simulink model "original"  (R2018a)
settings: Solver=VariableStepAuto  StartTime=0.0  StopTime=10.0  RelTol=1e-3
undefined symbols (not defined in the file): DiscIntNeverNeededParam, sigbuilder_block
libraries: simulink x479
(part 1 of 9)
settings Model: Creator=cyfuzz  LastModifiedBy=ishaf
settings CodeAppCC: StateflowObjectComments=on

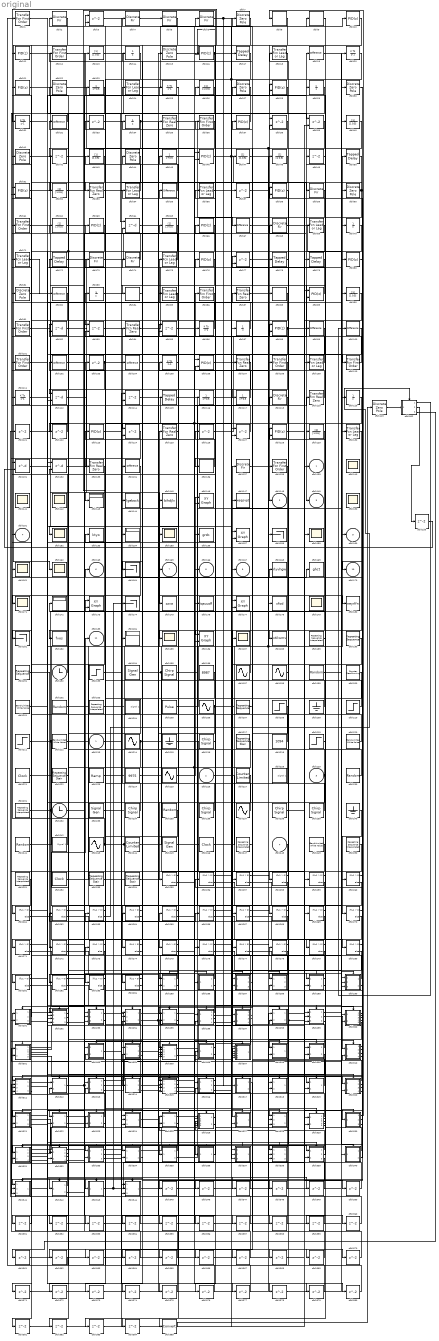
== system original ==
  cfblk213 : Inport
  cfblk226 : Inport  Port=2
  cfblk229 : Inport  Port=3
  cfblk248 : Inport  Port=4
  cfblk{1,12,36,61,86,91,101,108,110,138} (10 alike) : simulink/Discrete/Transfer Fcn First Order  PoleZ=0.95  ICPrevOutput=0.0  DoSatur=off
      settings: SourceProductName=Simulink
  cfblk{10..11,16,21,37,63,66,76,80,123} (10 alike) : simulink/Continuous/PID Controller  Controller=PID  TimeDomain=Discrete-time  SampleTime=1  IntegratorMethod=Forward Euler  FilterMethod=Forward Euler  Form=Parallel  UseFilter=on  ControllerParametersSource=internal  P=1  I=1  D=0  N=100  InitialConditionSource=internal  InitialConditionForIntegrator=0  InitialConditionForFilter=0  ExternalReset=none  LimitOutput=off  UpperSaturationLimit=inf  LowerSaturationLimit=-inf  LinearizeAsGain=off  AntiWindupMode=none  Kb=1  TrackingMode=off  Kt=1  PParamMin=[]  PParamMax=[]  IParamMin=[]  IParamMax=[]  DParamMin=[]  DParamMax=[]  NParamMin=[]  NParamMax=[]  KbParamMin=[]  KbParamMax=[]  KtParamMin=[]  KtParamMax=[]  POutMin=[]  POutMax=[]  IOutMin=[]  IOutMax=[]  DOutMin=[]  DOutMax=[]  NOutMin=[]  NOutMax=[]  KbOutMin=[]  KbOutMax=[]  KtOutMin=[]  KtOutMax=[]  IntegratorOutMin=[]  IntegratorOutMax=[]  FilterOutMin=[]  FilterOutMax=[]  SumOutMin=[]  SumOutMax=[]  SumI1OutMin=[]  SumI1OutMax=[]  SumI2OutMin=[]  SumI2OutMax=[]  SumI3OutMin=[]  SumI3OutMax=[]  SumDOutMin=[]  SumDOutMax=[]  SaturationOutMin=[]  SaturationOutMax=[]  IntegratorContinuousStateAttributes=''  IntegratorStateMustResolveToSignalObject=off  IntegratorRTWStateStorageClass=Auto  FilterContinuousStateAttributes=''  FilterStateMustResolveToSignalObject=off  FilterRTWStateStorageClass=Auto  DifferentiatorICPrevScaledInput=0  DifferentiatorOutMin=[]  DifferentiatorOutMax=[]  FilterDiffOutCoefMin=[]  FilterDiffOutCoefMax=[]  SumDenOutMin=[]  SumDenOutMax=[]  SumNumOutMin=[]  SumNumOutMax=[]  ReciprocalOutMin=[]  ReciprocalOutMax=[]  DivideOutMin=[]  DivideOutMax=[]  TunerSelectOption=Transfer Function Based (PID Tuner App)
  cfblk{19,32,55,67,82,99..100,102,104,134} (10 alike) : simulink/Discrete/Difference  ICPrevInput=0.0  OutMin=[]  OutMax=[]  OutDataTypeStr=Inherit: Inherit via back propagation  OutDataType=fixdt(1, 16)  OutScaling=2^-10  DoSatur=off
  cfblk{33,42,49,57,103,121..122,126,135,345..384} (49 alike) : Delay  SampleTime=1
  cfblk{20,25,31,96,105,111} (6 alike) : DiscreteIntegrator  ICPrevOutput=DiscIntNeverNeededParam  ICPrevScaledInput=DiscIntNeverNeededParam
  cfblk{28,46,51,58,89,98,106,128} (8 alike) : simulink/Continuous/PID Controller (2DOF)  Controller=PID  TimeDomain=Discrete-time  SampleTime=1  IntegratorMethod=Forward Euler  FilterMethod=Forward Euler  Form=Parallel  UseFilter=on  ControllerParametersSource=internal  P=1  I=1  D=0  N=100  b=1  c=1  InitialConditionSource=internal  InitialConditionForIntegrator=0  InitialConditionForFilter=0  ExternalReset=none  LimitOutput=off  UpperSaturationLimit=inf  LowerSaturationLimit=-inf  LinearizeAsGain=off  AntiWindupMode=none  Kb=1  TrackingMode=off  Kt=1  PParamMin=[]  PParamMax=[]  IParamMin=[]  IParamMax=[]  DParamMin=[]  DParamMax=[]  NParamMin=[]  NParamMax=[]  bParamMin=[]  bParamMax=[]  cParamMin=[]  cParamMax=[]  KbParamMin=[]  KbParamMax=[]  KtParamMin=[]  KtParamMax=[]  POutMin=[]  POutMax=[]  IOutMin=[]  IOutMax=[]  DOutMin=[]  DOutMax=[]  NOutMin=[]  NOutMax=[]  bOutMin=[]  bOutMax=[]  cOutMin=[]  cOutMax=[]  KbOutMin=[]  KbOutMax=[]  KtOutMin=[]  KtOutMax=[]  IntegratorOutMin=[]  IntegratorOutMax=[]  FilterOutMin=[]  FilterOutMax=[]  SumOutMin=[]  SumOutMax=[]  Sum1OutMin=[]  Sum1OutMax=[]  Sum2OutMin=[]  Sum2OutMax=[]  Sum3OutMin=[]  Sum3OutMax=[]  SumI1OutMin=[]  SumI1OutMax=[]  SumI2OutMin=[]  SumI2OutMax=[]  SumI3OutMin=[]  SumI3OutMax=[]  SumDOutMin=[]  SumDOutMax=[]  SaturationOutMin=[]  SaturationOutMax=[]  IntegratorContinuousStateAttributes=''  IntegratorStateMustResolveToSignalObject=off  IntegratorRTWStateStorageClass=Auto  FilterContinuousStateAttributes=''  FilterStateMustResolveToSignalObject=off  FilterRTWStateStorageClass=Auto  DifferentiatorICPrevScaledInput=0  DifferentiatorOutMin=[]  DifferentiatorOutMax=[]  FilterDiffOutCoefMin=[]  FilterDiffOutCoefMax=[]  SumDenOutMin=[]  SumDenOutMax=[]  SumNumOutMin=[]  SumNumOutMax=[]  ReciprocalOutMin=[]  ReciprocalOutMax=[]  DivideOutMin=[]  DivideOutMax=[]  TunerSelectOption=Transfer Function Based (PID Tuner App)
  cfblk{35,53,87,94,107,119,125,133} (8 alike) : simulink/Discrete/Transfer Fcn Real Zero  ZeroZ=0.75  ICPrevInput=0.0  DoSatur=off
      settings: SourceProductName=Simulink  SourceProductBaseCode=SL
  cfblk{18,24,54,56,69,71,75,85,109,130} (10 alike) : simulink/Discrete/Transfer Fcn Lead or Lag  PoleZ=0.95  ZeroZ=0.75  ICPrevOutput=0.0  ICPrevInput=0.0  DoSatur=off
      settings: SourceProductName=Simulink  SourceProductBaseCode=SL
  cfblk{64,92,112,131..132} (5 alike) : Delay  DelayLengthSource=Input port  SampleTime=1
      settings: InputPortMap=u0,p1
  cfblk{7,15,22,27,30,41,44,60,81,113} (10 alike) : DiscreteZeroPole  Poles=[0 0.5]  Gain=1
  cfblk{3,38..39,77,93,95,114,124,127} (9 alike) : Delay  ShowEnablePort=on  SampleTime=1
      settings: InputPortMap=u0,e6
  cfblk{17,50,72,78..79,115} (6 alike) : simulink/Discrete/Tapped Delay  vinit=0.0  samptime=-1  NumDelays=1  DelayOrder=Oldest  includeCurrent=off
  cfblk{23,45,116..117} (4 alike) : DiscreteTransferFcn  SampleTime=1
  cfblk{2,4..6,59,68,73..74,118,137} (10 alike) : DiscreteFir  SampleTime=1
  cfblk{14,29,34,70,83,97,120} (7 alike) : UnitDelay
  cfblk{13,26,40,43,47..48,52,62,65,90,129} (11 alike) : DiscreteFilter  SampleTime=1
  cfblk{8..9,84,88,136} (5 alike) : DiscreteStateSpace
  cfblk{140..142,150,152,155,159,161..162,171,179,185,187} (13 alike) : Scope
      cfblk140 settings: Floating=on
      cfblk141 settings: Floating=on
      cfblk142 settings: Floating=on
      cfblk150 settings: Floating=on
      cfblk179 settings: Floating=on
  cfblk{143,154,172,184} (4 alike) : Display
  cfblk144 : ToWorkspace  VariableName=lgebsck  SaveFormat=Timeseries  SampleTime=-1
  cfblk145 : ToWorkspace  VariableName=bihdjlv  SaveFormat=Timeseries  SampleTime=-1
  cfblk{146,157,173,177,186} (5 alike) : simulink/Sinks/XY Graph  xmin=-1  xmax=1  ymin=-1  ymax=1  st=-1
  cfblk147 : ToWorkspace  VariableName=xeqpvpt  SaveFormat=Timeseries  SampleTime=-1
  cfblk153 : ToFile  Filename=ktyo  SaveFormat=Timeseries
  cfblk156 : ToFile  Filename=grzb  SaveFormat=Timeseries
  cfblk{158,164,174,181} (4 alike) : Terminator
  cfblk168 : ToWorkspace  VariableName=rlyvhgw  SaveFormat=Timeseries  SampleTime=-1
  cfblk169 : ToFile  Filename=ghct  SaveFormat=Timeseries
  cfblk175 : ToFile  Filename=zzva  SaveFormat=Timeseries
  cfblk176 : ToWorkspace  VariableName=iqauudf  SaveFormat=Timeseries  SampleTime=-1
  cfblk178 : ToFile  Filename=xfod  SaveFormat=Timeseries
  cfblk180 : ToWorkspace  VariableName=neyrlfn  SaveFormat=Timeseries  SampleTime=-1
  cfblk182 : ToFile  Filename=fvos  SaveFormat=Timeseries
  cfblk188 : ToWorkspace  VariableName=xtilwmv  SaveFormat=Timeseries  SampleTime=-1
  cfblk{189,203,231,247,250..251} (6 alike) : simulink/Sources/Repeating Sequence Interpolated  OutValues=[3 1 4 2 1].'  TimeValues=[0 0.1 0.5 0.6 1].'  LookUpMeth=Interpolation-Use End Values  tsamp=0.01  OutMin=[]  OutMax=[]  OutDataTypeStr=double  OutputDataTypeScalingMode=double  OutDataType=fixdt(0,8)  OutScaling=2^-10
  cfblk190 : simulink/Sources/Repeating Sequence  rep_seq_t=[0 2]  rep_seq_y=[0 2]
  cfblk191 : simulink/Sources/Repeating Sequence  rep_seq_t=[0 2]  rep_seq_y=[0 2]
  cfblk192 : Clock
  cfblk193 : Step  After=18  SampleTime=0
  cfblk194 : SignalGenerator  Units=rad/sec
  cfblk{195,216,234,236,238..239} (6 alike) : simulink/Sources/Chirp Signal  f1=0.1  T=100  f2=1
  cfblk196 : Constant  Value=8987
  cfblk{197..198,206,214,225,237,243} (7 alike) : Sin  SampleTime=0
  cfblk{199,230,235,241} (4 alike) : RandomNumber  SampleTime=0.1
  cfblk200 : simulink/Sources/Counter Free-Running  NumBits=16  tsamp=-1
  cfblk{201,212,220,249} (4 alike) : simulink/Sources/Band-Limited White Noise  Cov=[0.1]  Ts=0.1  seed=[23341]
  cfblk202 : UniformRandomNumber  SampleTime=0.1
  cfblk204 : Subsystem  Tag=STV Subsys  LoadFcn=sigbuilder_block('load');  StartFcn=sigbuilder_block('start');  StopFcn=sigbuilder_block('stop');  ClipboardFcn=sigbuilder_block('clipboard');  mask(Sigbuilder block){tuvar=[0:10]}
      mask help: Simulink:masks:SigbuilderBlock_MD
      mask init:
      | if ~strcmp(get_param(bdroot(gcbh),'SimulationStatus'),'stopped') tuvar = sigbuilder_block('maskInit'); end
      settings: CopyFcn=sigbuilder_block('copy');  DeleteFcn=sigbuilder_block('delete');  ModelCloseFcn=sigbuilder_block('modelClose');  PreSaveFcn=sigbuilder_block('preSave');  PauseFcn=sigbuilder_block('pause');  ContinueFcn=sigbuilder_block('continue');  NameChangeFcn=sigbuilder_block('namechange');  OpenFcn=sigbuilder_block('open',[437.6 199.2 550.4 400 ]);  CloseFcn=sigbuilder_block('close');
      mask Display: plot(0, 0, 100, 100,[2, 2, 32, 32, 2], [68, 8, 8, 68, 68],[32, 2], [38, 38], [32, 19, 2],[53, 60, 44], [32, 17, 17, 2],[16, 16, 31, 31]);txt = getActiveGroup(gcbh);text(2, 100, txt,'verticalAlignment', 'top');
  cfblk205 : DiscretePulseGenerator  PulseType=Time based  Period=10  PulseWidth=5
  cfblk207 : simulink/Sources/Repeating Sequence  rep_seq_t=[0 2]  rep_seq_y=[0 2]
  cfblk208 : Step  After=83  SampleTime=0
  cfblk209 : Ground
  cfblk210 : Step  After=27  SampleTime=0
  cfblk211 : Step  After=11  SampleTime=0
  cfblk215 : Ground
  cfblk{217,222,253..254} (4 alike) : simulink/Sources/Repeating Sequence Stair  OutValues=[3 1 4 2 1].'  tsamp=-1  OutMin=[]  OutMax=[]  OutDataTypeStr=double  OutputDataTypeScalingMode=double  OutDataType=fixdt(0,8)  ConRadixGroup=Best Precision: Vector-wise  OutScaling=2^-12
  cfblk218 : Constant  Value=1094
  cfblk219 : Step  After=49  SampleTime=0
  cfblk221 : DigitalClock
  cfblk223 : simulink/Sources/Ramp  slope=1  start=0  InitialOutput=0
  cfblk224 : Constant  Value=9975
  cfblk227 : simulink/Sources/Counter Limited  uplimit=7  tsamp=-1
  cfblk228 : Subsystem  Tag=STV Subsys  LoadFcn=sigbuilder_block('load');  StartFcn=sigbuilder_block('start');  StopFcn=sigbuilder_block('stop');  ClipboardFcn=sigbuilder_block('clipboard');  mask(Sigbuilder block){tuvar=[0:10]}
      mask help: Simulink:masks:SigbuilderBlock_MD
      mask init:
      | if ~strcmp(get_param(bdroot(gcbh),'SimulationStatus'),'stopped') tuvar = sigbuilder_block('maskInit'); end
      settings: CopyFcn=sigbuilder_block('copy');  DeleteFcn=sigbuilder_block('delete');  ModelCloseFcn=sigbuilder_block('modelClose');  PreSaveFcn=sigbuilder_block('preSave');  PauseFcn=sigbuilder_block('pause');  ContinueFcn=sigbuilder_block('continue');  NameChangeFcn=sigbuilder_block('namechange');  OpenFcn=sigbuilder_block('open',[437.6 199.2 550.4 400 ]);  CloseFcn=sigbuilder_block('close');
      mask Display: plot(0, 0, 100, 100,[2, 2, 32, 32, 2], [68, 8, 8, 68, 68],[32, 2], [38, 38], [32, 19, 2],[53, 60, 44], [32, 17, 17, 2],[16, 16, 31, 31]);txt = getActiveGroup(gcbh);text(2, 100, txt,'verticalAlignment', 'top');
  cfblk232 : Clock
  cfblk233 : SignalGenerator  Units=rad/sec
  cfblk240 : Ground
  cfblk242 : Subsystem  Tag=STV Subsys  LoadFcn=sigbuilder_block('load');  StartFcn=sigbuilder_block('start');  StopFcn=sigbuilder_block('stop');  ClipboardFcn=sigbuilder_block('clipboard');  mask(Sigbuilder block){tuvar=[0:10]}
      mask help: Simulink:masks:SigbuilderBlock_MD
      mask init:
      | if ~strcmp(get_param(bdroot(gcbh),'SimulationStatus'),'stopped') tuvar = sigbuilder_block('maskInit'); end
      settings: CopyFcn=sigbuilder_block('copy');  DeleteFcn=sigbuilder_block('delete');  ModelCloseFcn=sigbuilder_block('modelClose');  PreSaveFcn=sigbuilder_block('preSave');  PauseFcn=sigbuilder_block('pause');  ContinueFcn=sigbuilder_block('continue');  NameChangeFcn=sigbuilder_block('namechange');  OpenFcn=sigbuilder_block('open',[437.6 199.2 550.4 400 ]);  CloseFcn=sigbuilder_block('close');
      mask Display: plot(0, 0, 100, 100,[2, 2, 32, 32, 2], [68, 8, 8, 68, 68],[32, 2], [38, 38], [32, 19, 2],[53, 60, 44], [32, 17, 17, 2],[16, 16, 31, 31]);txt = getActiveGroup(gcbh);text(2, 100, txt,'verticalAlignment', 'top');
  cfblk244 : simulink/Sources/Counter Limited  uplimit=7  tsamp=-1
  cfblk245 : SignalGenerator  Units=rad/sec
  cfblk246 : DigitalClock
  cfblk252 : DigitalClock
  cfblk{255..284} (30 alike) : If  SampleTime=1
  cfblk285 : Subsystem  TreatAsAtomicUnit=on
  cfblk286 : Subsystem  TreatAsAtomicUnit=on
  cfblk287 : Subsystem  TreatAsAtomicUnit=on
  cfblk288 : Subsystem  TreatAsAtomicUnit=on
  cfblk289 : Subsystem  TreatAsAtomicUnit=on
  cfblk290 : Subsystem  TreatAsAtomicUnit=on
  cfblk291 : Subsystem  TreatAsAtomicUnit=on
  cfblk292 : Subsystem  TreatAsAtomicUnit=on
  cfblk293 : Subsystem  TreatAsAtomicUnit=on
  cfblk294 : Subsystem  TreatAsAtomicUnit=on
  cfblk295 : Subsystem  TreatAsAtomicUnit=on
  cfblk296 : Subsystem  TreatAsAtomicUnit=on
  cfblk297 : Subsystem  TreatAsAtomicUnit=on
  cfblk298 : Subsystem  TreatAsAtomicUnit=on
  cfblk299 : Subsystem  TreatAsAtomicUnit=on
  cfblk300 : Subsystem  TreatAsAtomicUnit=on
  cfblk301 : Subsystem  TreatAsAtomicUnit=on
  cfblk302 : Subsystem  TreatAsAtomicUnit=on
  cfblk303 : Subsystem  TreatAsAtomicUnit=on
  cfblk304 : Subsystem  TreatAsAtomicUnit=on
  cfblk305 : Subsystem  TreatAsAtomicUnit=on
  cfblk306 : Subsystem  TreatAsAtomicUnit=on
  cfblk307 : Subsystem  TreatAsAtomicUnit=on
  cfblk308 : Subsystem  TreatAsAtomicUnit=on
  cfblk309 : Subsystem  TreatAsAtomicUnit=on
  cfblk310 : Subsystem  TreatAsAtomicUnit=on
  cfblk311 : Subsystem  TreatAsAtomicUnit=on
  cfblk312 : Subsystem  TreatAsAtomicUnit=on
  cfblk313 : Subsystem  TreatAsAtomicUnit=on
  cfblk314 : Subsystem  TreatAsAtomicUnit=on
  cfblk315 : Subsystem  TreatAsAtomicUnit=on
  cfblk316 : Subsystem  TreatAsAtomicUnit=on
  cfblk317 : Subsystem  TreatAsAtomicUnit=on
  cfblk318 : Subsystem  TreatAsAtomicUnit=on
  cfblk319 : Subsystem  TreatAsAtomicUnit=on
  cfblk320 : Subsystem  TreatAsAtomicUnit=on
  cfblk321 : Subsystem  TreatAsAtomicUnit=on
  cfblk322 : Subsystem  TreatAsAtomicUnit=on
  cfblk323 : Subsystem  TreatAsAtomicUnit=on
  cfblk324 : Subsystem  TreatAsAtomicUnit=on
  cfblk325 : Subsystem  TreatAsAtomicUnit=on
  cfblk326 : Subsystem  TreatAsAtomicUnit=on
  cfblk327 : Subsystem  TreatAsAtomicUnit=on
  cfblk328 : Subsystem  TreatAsAtomicUnit=on
  cfblk329 : Subsystem  TreatAsAtomicUnit=on
  cfblk330 : Subsystem  TreatAsAtomicUnit=on
  cfblk331 : Subsystem  TreatAsAtomicUnit=on
  cfblk332 : Subsystem  TreatAsAtomicUnit=on
  cfblk333 : Subsystem  TreatAsAtomicUnit=on
  cfblk334 : Subsystem  TreatAsAtomicUnit=on
  cfblk335 : Subsystem  TreatAsAtomicUnit=on
  cfblk336 : Subsystem  TreatAsAtomicUnit=on
  cfblk337 : Subsystem  TreatAsAtomicUnit=on
  cfblk338 : Subsystem  TreatAsAtomicUnit=on
  cfblk339 : Subsystem  TreatAsAtomicUnit=on
  cfblk340 : Subsystem  TreatAsAtomicUnit=on
  cfblk341 : Subsystem  TreatAsAtomicUnit=on
  cfblk342 : Subsystem  TreatAsAtomicUnit=on
  cfblk343 : Subsystem  TreatAsAtomicUnit=on
  cfblk344 : Subsystem  TreatAsAtomicUnit=on
  cfblk385 : DataTypeConversion
  cfblk139 : Outport
  cfblk148 : Outport  Port=2
  cfblk149 : Outport  Port=3
  cfblk151 : Outport  Port=4
  cfblk160 : Outport  Port=5
  cfblk163 : Outport  Port=6
  cfblk165 : Outport  Port=7
  cfblk166 : Outport  Port=8
  cfblk167 : Outport  Port=9
  cfblk170 : Outport  Port=10
  cfblk183 : Outport  Port=11
  wires:
  cfblk73/1 -> cfblk65/1
  cfblk79/1 -> cfblk149/1
  cfblk115/1 -> cfblk268/1
  cfblk249/1 -> cfblk265/1
  cfblk24/1 -> cfblk6/1
  cfblk331/1(cfblk2) -> cfblk119/1
  cfblk61/1 -> cfblk143/1
  cfblk189/1 -> cfblk13/1
  cfblk223/1 -> cfblk50/1
  cfblk2/1 -> cfblk162/1
  cfblk15/1 -> cfblk274/1
  cfblk10/1 -> cfblk148/1
  cfblk225/1 -> cfblk146/1
  cfblk252/1 -> cfblk125/1
  cfblk342/1(cfblk2) -> cfblk291/1(cfblk1)
  cfblk215/1 -> cfblk318/1(cfblk1)
  cfblk305/1(cfblk2) -> cfblk137/1
  cfblk242/1(Signal 1) -> cfblk16/1
  cfblk129/1 -> cfblk327/1(cfblk1)
  cfblk128/1 -> cfblk269/1
  cfblk117/1 -> cfblk34/1
  cfblk92/1 -> cfblk175/1
  cfblk296/1(cfblk2) -> cfblk105/1
  cfblk319/1(cfblk2) -> cfblk264/1
  cfblk323/1(cfblk2) -> cfblk183/1
  cfblk305/2(cfblk13) -> cfblk57/1
  cfblk122/1 -> cfblk11/1
  cfblk240/1 -> cfblk270/1
  cfblk37/1 -> cfblk64/1
  cfblk316/1(cfblk2) -> cfblk121/1
  cfblk325/1(cfblk2) -> cfblk70/1
  cfblk293/1(cfblk2) -> cfblk330/1(cfblk1)
  cfblk46/1 -> cfblk299/1(cfblk1), cfblk339/2(cfblk13)
  cfblk47/1 -> cfblk108/1
  cfblk314/1(cfblk2) -> cfblk103/1
  cfblk63/1 -> cfblk342/1(cfblk1)
  cfblk102/1 -> cfblk74/1
  cfblk67/1 -> cfblk138/1
  cfblk71/1 -> cfblk82/1
  cfblk241/1 -> cfblk48/1
  cfblk224/1 -> cfblk106/1
  cfblk238/1 -> cfblk329/1(cfblk1)
  cfblk235/1 -> cfblk343/1(cfblk1)
  cfblk49/1 -> cfblk319/1(cfblk1)
  cfblk72/1 -> cfblk318/2(cfblk11)
  cfblk228/1(Signal 1) -> cfblk26/1
  cfblk197/1 -> cfblk172/1
  cfblk5/1 -> cfblk334/1(cfblk1)
  cfblk193/1 -> cfblk324/1(cfblk1)
  cfblk246/1 -> cfblk30/1
  cfblk199/1 -> cfblk20/1
  cfblk54/1 -> cfblk43/1
  cfblk97/1 -> cfblk75/1
  cfblk196/1 -> cfblk333/1(cfblk1)
  cfblk51/1 -> cfblk25/1
  cfblk22/1 -> cfblk316/1(cfblk1)
  cfblk127/1 -> cfblk45/1
  cfblk132/1 -> cfblk78/1
  cfblk331/2(cfblk10) -> cfblk323/1(cfblk1)
  cfblk7/1 -> cfblk181/1
  cfblk336/1(cfblk2) -> cfblk66/1
  cfblk58/1 -> cfblk288/1(cfblk1)
  cfblk13/1 -> cfblk38/1
  cfblk291/1(cfblk2) -> cfblk120/1
  cfblk59/1 -> cfblk308/1(cfblk1)
  cfblk209/1 -> cfblk58/1
  cfblk35/1 -> cfblk67/1
  cfblk121/1 -> cfblk19/1
  cfblk237/1 -> cfblk73/1
  cfblk307/1(cfblk2) -> cfblk166/1
  cfblk82/1 -> cfblk271/1
  cfblk95/1 -> cfblk86/1
  cfblk109/1 -> cfblk32/1
  cfblk243/1 -> cfblk177/2, cfblk307/5(cfblk15), cfblk81/1
  cfblk65/1 -> cfblk281/1
  cfblk85/1 -> cfblk182/1
  cfblk302/1(cfblk2) -> cfblk100/1
  cfblk310/1(cfblk2) -> cfblk60/1
  cfblk218/1 -> cfblk55/1
  cfblk39/1 -> cfblk297/1(cfblk1)
  cfblk41/1 -> cfblk303/1(cfblk1)
  cfblk247/1 -> cfblk87/1
  cfblk20/1 -> cfblk283/1, cfblk337/3(cfblk13)
  cfblk324/1(cfblk2) -> cfblk35/1
  cfblk244/1 -> cfblk156/1
  cfblk114/1 -> cfblk286/1(cfblk1)
  cfblk190/1 -> cfblk277/1
  cfblk96/1 -> cfblk61/1
  cfblk194/1 -> cfblk308/2(cfblk10), cfblk128/2
  cfblk308/1(cfblk2) -> cfblk24/1
  cfblk191/1 -> cfblk272/1
  cfblk300/2(cfblk13) -> cfblk311/1(cfblk1)
  cfblk212/1 -> cfblk324/2(cfblk8)
  cfblk206/1 -> cfblk88/1, cfblk305/5(cfblk12)
  cfblk48/1 -> cfblk284/1
  cfblk217/1 -> cfblk322/1(cfblk1), cfblk326/4(cfblk8)
  cfblk339/1(cfblk2) -> cfblk325/1(cfblk1)
  cfblk130/1 -> cfblk275/1
  cfblk8/1 -> cfblk186/1
  cfblk75/1 -> cfblk51/1
  cfblk69/1 -> cfblk122/1, cfblk292/3(cfblk14)
  cfblk298/1(cfblk2) -> cfblk89/1
  cfblk211/1 -> cfblk146/2, cfblk305/4(cfblk11)
  cfblk219/1 -> cfblk279/1
  cfblk94/1 -> cfblk40/1
  cfblk321/1(cfblk2) -> cfblk90/1
  cfblk214/1 -> cfblk97/1, cfblk292/1(cfblk1)
  cfblk210/1 -> cfblk63/1
  cfblk302/2(cfblk13) -> cfblk135/1
  cfblk314/2(cfblk8) -> cfblk160/1
  cfblk80/1 -> cfblk170/1
  cfblk126/1 -> cfblk89/2
  cfblk329/1(cfblk2) -> cfblk304/2(cfblk7)
  cfblk118/1 -> cfblk186/2, cfblk373/1
  cfblk335/1(cfblk2) -> cfblk44/1
  cfblk248/1 -> cfblk332/1(cfblk1)
  cfblk310/2(cfblk14) -> cfblk256/1
  cfblk108/1 -> cfblk112/1
  cfblk290/1(cfblk2) -> cfblk151/1
  cfblk231/1 -> cfblk116/1, cfblk315/4(cfblk10)
  cfblk98/1 -> cfblk292/2(cfblk13), cfblk350/1
  cfblk297/1(cfblk2) -> cfblk83/1
  cfblk66/1 -> cfblk93/1
  cfblk33/1 -> cfblk59/1
  cfblk330/1(cfblk2) -> cfblk8/1
  cfblk32/1 -> cfblk31/1
  cfblk104/1 -> cfblk180/1
  cfblk195/1 -> cfblk99/1, cfblk98/2
  cfblk74/1 -> cfblk21/1
  cfblk328/1(cfblk2) -> cfblk56/1
  cfblk27/1 -> cfblk291/2(cfblk7)
  cfblk301/1(cfblk2) -> cfblk139/1
  cfblk289/1(cfblk2) -> cfblk301/2(cfblk12)
  cfblk251/1 -> cfblk261/1
  cfblk233/1 -> cfblk79/1
  cfblk234/1 -> cfblk94/1
  cfblk44/1 -> cfblk133/1
  cfblk119/1 -> cfblk18/1
  cfblk227/1 -> cfblk255/1
  cfblk230/1 -> cfblk104/1
  cfblk232/1 -> cfblk313/1(cfblk1)
  cfblk288/1(cfblk2) -> cfblk64/2
  cfblk38/1 -> cfblk333/2(cfblk15), cfblk328/3(cfblk8)
  cfblk298/2(cfblk9) -> cfblk159/1, cfblk28/2
  cfblk310/3(cfblk15) -> cfblk288/2(cfblk7)
  cfblk343/1(cfblk2) -> cfblk259/1, cfblk174/1
  cfblk310/4(cfblk16) -> cfblk161/1
  cfblk26/1 -> cfblk42/1
  cfblk332/2(cfblk10) -> cfblk62/1
  cfblk42/1 -> cfblk290/3(cfblk10)
  cfblk89/1 -> cfblk84/1
  cfblk29/1 -> cfblk152/1
  cfblk293/2(cfblk12) -> cfblk102/1
  cfblk330/2(cfblk13) -> cfblk165/1
  cfblk220/1 -> cfblk91/1
  cfblk340/1(cfblk2) -> cfblk278/1
  cfblk107/1 -> cfblk117/1
  cfblk216/1 -> cfblk36/1
  cfblk309/1(cfblk2) -> cfblk37/1
  cfblk328/2(cfblk9) -> cfblk147/1
  cfblk332/3(cfblk11) -> cfblk331/1(cfblk1)
  cfblk208/1 -> cfblk287/1(cfblk1)
  cfblk125/1 -> cfblk155/1
  cfblk296/2(cfblk12) -> cfblk338/1(cfblk1)
  cfblk198/1 -> cfblk68/1
  cfblk335/2(cfblk11) -> cfblk157/1
  cfblk68/1 -> cfblk260/1
  cfblk290/2(cfblk11) -> cfblk96/1
  cfblk312/1(cfblk2) -> cfblk307/3(cfblk13), cfblk355/1
  cfblk88/1 -> cfblk341/1(cfblk1)
  cfblk331/3(cfblk11) -> cfblk154/1
  cfblk78/1 -> cfblk38/2
  cfblk133/1 -> cfblk321/1(cfblk1)
  cfblk84/1 -> cfblk14/1
  cfblk103/1 -> cfblk307/6(cfblk16), cfblk372/1
  cfblk207/1 -> cfblk7/1
  cfblk57/1 -> cfblk158/1
  cfblk11/1 -> cfblk293/3(cfblk11)
  cfblk323/2(cfblk17) -> cfblk2/1
  cfblk93/1 -> cfblk307/1(cfblk1)
  cfblk301/2(cfblk13) -> cfblk187/1
  cfblk338/1(cfblk2) -> cfblk316/2(cfblk9)
  cfblk192/1 -> cfblk71/1
  cfblk221/1 -> cfblk114/1
  cfblk332/4(cfblk12) -> cfblk266/1
  cfblk113/1 -> cfblk302/1(cfblk1)
  cfblk330/3(cfblk14) -> cfblk168/1
  cfblk101/1 -> cfblk323/2(cfblk16)
  cfblk116/1 -> cfblk9/1
  cfblk30/1 -> cfblk320/1(cfblk1)
  cfblk34/1 -> cfblk145/1, cfblk344/3(cfblk13)
  cfblk203/1 -> cfblk46/1
  cfblk23/1 -> cfblk51/2
  cfblk285/1(cfblk2) -> cfblk33/1
  cfblk12/1 -> cfblk305/1(cfblk1)
  cfblk306/1(cfblk2) -> cfblk335/1(cfblk1)
  cfblk320/1(cfblk2) -> cfblk12/1
  cfblk81/1 -> cfblk157/2
  cfblk14/1 -> cfblk53/1
  cfblk70/1 -> cfblk124/1
  cfblk294/1(cfblk2) -> cfblk296/2(cfblk11)
  cfblk300/3(cfblk14) -> cfblk58/2
  cfblk301/3(cfblk14) -> cfblk76/1
  cfblk344/1(cfblk2) -> cfblk309/1(cfblk1)
  cfblk40/1 -> cfblk46/2
  cfblk333/1(cfblk2) -> cfblk124/2
  cfblk138/1 -> cfblk188/1
  cfblk331/4(cfblk12) -> cfblk184/1
  cfblk325/2(cfblk7) -> cfblk144/1
  cfblk45/1 -> cfblk289/1(cfblk1)
  cfblk287/1(cfblk2) -> cfblk131/1
  cfblk87/1 -> cfblk280/1
  cfblk303/1(cfblk2) -> cfblk169/1
  cfblk137/1 -> cfblk178/1
  cfblk288/2(cfblk8) -> cfblk92/1
  cfblk288/3(cfblk9) -> cfblk93/2
  cfblk286/1(cfblk2) -> cfblk101/1
  cfblk287/2(cfblk13) -> cfblk95/1
  cfblk311/1(cfblk2) -> cfblk27/1
  cfblk110/1 -> cfblk72/1
  cfblk131/1 -> cfblk276/1
  cfblk297/2(cfblk5) -> cfblk295/1(cfblk1)
  cfblk21/1 -> cfblk167/1
  cfblk326/2(cfblk10) -> cfblk153/1
  cfblk311/2(cfblk12) -> cfblk306/1(cfblk1)
  cfblk342/2(cfblk10) -> cfblk69/1
  cfblk91/1 -> cfblk326/1(cfblk1)
  cfblk16/1 -> cfblk337/1(cfblk1), cfblk314/1(cfblk1)
  cfblk340/2(cfblk13) -> cfblk287/2(cfblk12)
  cfblk285/2(cfblk12) -> cfblk54/1
  cfblk299/1(cfblk2) -> cfblk80/1
  cfblk229/1 -> cfblk92/2, cfblk292/4(cfblk15)
  cfblk112/1 -> cfblk15/1
  cfblk202/1 -> cfblk267/1
  cfblk299/2(cfblk14) -> cfblk310/1(cfblk1)
  cfblk304/1(cfblk2) -> cfblk173/1
  cfblk55/1 -> cfblk23/1
  cfblk318/1(cfblk2) -> cfblk77/1
  cfblk222/1 -> cfblk22/1
  cfblk111/1 -> cfblk344/1(cfblk1)
  cfblk136/1 -> cfblk123/1
  cfblk17/1 -> cfblk344/2(cfblk12)
  cfblk245/1 -> cfblk289/2(cfblk6)
  cfblk297/3(cfblk6) -> cfblk4/1
  cfblk56/1 -> cfblk110/1
  cfblk18/1 -> cfblk164/1
  cfblk25/1 -> cfblk185/1
  cfblk320/2(cfblk13) -> cfblk310/2(cfblk13)
  cfblk294/2(cfblk14) -> cfblk115/1, cfblk307/4(cfblk14)
  cfblk315/1(cfblk2) -> cfblk307/2(cfblk12)
  cfblk334/1(cfblk2) -> cfblk118/1
  cfblk201/1 -> cfblk112/2
  cfblk289/2(cfblk7) -> cfblk176/1
  cfblk316/2(cfblk10) -> cfblk47/1
  cfblk60/1 -> cfblk52/1, cfblk326/5(cfblk9)
  cfblk316/3(cfblk11) -> cfblk17/1
  cfblk52/1 -> cfblk28/1
  cfblk236/1 -> cfblk3/1
  cfblk327/1(cfblk2) -> cfblk111/1
  cfblk291/2(cfblk8) -> cfblk41/1
  cfblk239/1 -> cfblk126/1
  cfblk338/2(cfblk8) -> cfblk106/2
  cfblk292/1(cfblk2) -> cfblk331/2(cfblk9)
  cfblk314/3(cfblk9) -> cfblk130/1
  cfblk286/2(cfblk10) -> cfblk134/1
  cfblk205/1 -> cfblk109/1
  cfblk295/2(cfblk11) -> cfblk173/2
  cfblk254/1 -> cfblk328/1(cfblk1)
  cfblk226/1 -> cfblk258/1
  cfblk299/3(cfblk15) -> cfblk128/1
  cfblk253/1 -> cfblk300/1(cfblk1)
  cfblk120/1 -> cfblk336/1(cfblk1)
  cfblk1/1 -> cfblk39/1
  cfblk135/1 -> cfblk131/2
  cfblk306/2(cfblk12) -> cfblk3/2
  cfblk301/4(cfblk15) -> cfblk294/3(cfblk13)
  cfblk76/1 -> cfblk324/3(cfblk9)
  cfblk250/1 -> cfblk311/4(cfblk11)
  cfblk300/4(cfblk15) -> cfblk341/2(cfblk15)
  cfblk313/1(cfblk2) -> cfblk95/2
  cfblk329/3(cfblk12) -> cfblk338/2(cfblk6)
  cfblk19/1 -> cfblk300/2(cfblk12)
  cfblk4/1 -> cfblk5/1
  cfblk83/1 -> cfblk127/2
  cfblk90/1 -> cfblk309/2(cfblk13)
  cfblk296/3(cfblk13) -> cfblk262/1
  cfblk296/4(cfblk14) -> cfblk327/2(cfblk11)
  cfblk322/2(cfblk12) -> cfblk98/1
  cfblk292/3(cfblk17) -> cfblk85/1
  cfblk31/1 -> cfblk29/1
  cfblk320/3(cfblk14) -> cfblk329/2(cfblk10)
  cfblk321/2(cfblk7) -> cfblk339/1(cfblk1)
  cfblk134/1 -> cfblk171/1
  cfblk301/5(cfblk16) -> cfblk320/2(cfblk12)
  cfblk124/1 -> cfblk341/3(cfblk16)
  cfblk6/1 -> cfblk107/1, cfblk317/1(cfblk1)
  cfblk320/4(cfblk15) -> cfblk163/1
  cfblk99/1 -> cfblk285/1(cfblk1)
  cfblk213/1 -> cfblk114/2
  cfblk338/3(cfblk9) -> cfblk326/3(cfblk7)
  cfblk106/1 -> cfblk177/1
  cfblk339/2(cfblk14) -> cfblk49/1
  cfblk204/1(Signal 1) -> cfblk282/1
  cfblk329/5(cfblk14) -> cfblk77/2
  cfblk297/4(cfblk7) -> cfblk322/2(cfblk11)
  cfblk50/1 -> cfblk315/1(cfblk1)
  cfblk313/3(cfblk15) -> cfblk285/2(cfblk11)
  cfblk36/1 -> cfblk315/2(cfblk8)
  cfblk304/3(cfblk9) -> cfblk132/2
  cfblk9/1 -> cfblk129/1
  cfblk28/1 -> cfblk136/1
  cfblk315/2(cfblk11) -> cfblk332/2(cfblk9)
  cfblk315/4(cfblk13) -> cfblk10/1
  cfblk255/1 -> cfblk285/Action
  cfblk255/2 -> cfblk286/Action
  cfblk256/1 -> cfblk287/Action
  cfblk256/2 -> cfblk288/Action
  cfblk257/1 -> cfblk289/Action
  cfblk257/2 -> cfblk290/Action
  cfblk258/1 -> cfblk291/Action
  cfblk258/2 -> cfblk292/Action
  cfblk259/1 -> cfblk293/Action
  cfblk259/2 -> cfblk294/Action
  cfblk260/1 -> cfblk295/Action
  cfblk260/2 -> cfblk296/Action
  cfblk261/1 -> cfblk297/Action
  cfblk261/2 -> cfblk298/Action
  cfblk262/1 -> cfblk299/Action
  cfblk262/2 -> cfblk300/Action
  cfblk263/1 -> cfblk301/Action
  cfblk263/2 -> cfblk302/Action
  cfblk264/1 -> cfblk303/Action
  cfblk264/2 -> cfblk304/Action
  cfblk265/1 -> cfblk305/Action
  cfblk265/2 -> cfblk306/Action
  cfblk266/1 -> cfblk307/Action
  cfblk266/2 -> cfblk308/Action
  cfblk267/1 -> cfblk309/Action
  cfblk267/2 -> cfblk310/Action
  cfblk268/1 -> cfblk311/Action
  cfblk268/2 -> cfblk312/Action
  cfblk269/1 -> cfblk313/Action
  cfblk269/2 -> cfblk314/Action
  cfblk270/1 -> cfblk315/Action
  cfblk270/2 -> cfblk316/Action
  cfblk271/1 -> cfblk317/Action
  cfblk271/2 -> cfblk318/Action
  cfblk272/1 -> cfblk319/Action
  cfblk272/2 -> cfblk320/Action
  cfblk273/1 -> cfblk321/Action
  cfblk273/2 -> cfblk322/Action
  cfblk274/1 -> cfblk323/Action
  cfblk274/2 -> cfblk324/Action
  cfblk275/1 -> cfblk325/Action
  cfblk275/2 -> cfblk326/Action
  cfblk276/1 -> cfblk327/Action
  cfblk276/2 -> cfblk328/Action
  cfblk277/1 -> cfblk329/Action
  cfblk277/2 -> cfblk330/Action
  cfblk278/1 -> cfblk331/Action
  cfblk278/2 -> cfblk332/Action
  cfblk279/1 -> cfblk333/Action
  cfblk279/2 -> cfblk334/Action
  cfblk280/1 -> cfblk335/Action
  cfblk280/2 -> cfblk336/Action
  cfblk281/1 -> cfblk337/Action
  cfblk281/2 -> cfblk338/Action
  cfblk282/1 -> cfblk339/Action
  cfblk282/2 -> cfblk340/Action
  cfblk283/1 -> cfblk341/Action
  cfblk283/2 -> cfblk342/Action
  cfblk284/1 -> cfblk343/Action
  cfblk284/2 -> cfblk344/Action
  cfblk105/1 -> cfblk345/1
  cfblk345/1 -> cfblk39/2
  cfblk300/1(cfblk2) -> cfblk346/1
  cfblk346/1 -> cfblk290/2(cfblk9)
  cfblk291/3(cfblk9) -> cfblk347/1
  cfblk347/1 -> cfblk311/3(cfblk10)
  cfblk64/1 -> cfblk348/1
  cfblk348/1 -> cfblk273/1
  cfblk322/1(cfblk2) -> cfblk349/1
  cfblk349/1 -> cfblk296/1(cfblk1)
  cfblk350/1 -> cfblk301/1(cfblk1)
  cfblk292/2(cfblk16) -> cfblk351/1
  cfblk351/1 -> cfblk321/2(cfblk6)
  cfblk309/2(cfblk14) -> cfblk352/1
  cfblk352/1 -> cfblk294/2(cfblk12)
  cfblk341/1(cfblk2) -> cfblk353/1
  cfblk353/1 -> cfblk326/2(cfblk6)
  cfblk326/1(cfblk2) -> cfblk354/1
  cfblk354/1 -> cfblk312/1(cfblk1)
  cfblk355/1 -> cfblk325/2(cfblk6)
  cfblk304/2(cfblk8) -> cfblk356/1
  cfblk356/1 -> cfblk340/1(cfblk1)
  cfblk332/1(cfblk2) -> cfblk357/1
  cfblk357/1 -> cfblk303/2(cfblk9)
  cfblk62/1 -> cfblk358/1
  cfblk358/1 -> cfblk263/1
  cfblk100/1 -> cfblk359/1
  cfblk359/1 -> cfblk293/2(cfblk10)
  cfblk77/1 -> cfblk360/1
  cfblk360/1 -> cfblk328/2(cfblk7)
  cfblk302/3(cfblk14) -> cfblk361/1
  cfblk361/1 -> cfblk305/2(cfblk9)
  cfblk317/1(cfblk2) -> cfblk362/1
  cfblk362/1 -> cfblk1/1
  cfblk317/2(cfblk7) -> cfblk363/1
  cfblk363/1 -> cfblk337/2(cfblk12)
  cfblk337/1(cfblk2) -> cfblk364/1
  cfblk364/1 -> cfblk311/2(cfblk9)
  cfblk86/1 -> cfblk365/1
  cfblk365/1 -> cfblk293/1(cfblk1)
  cfblk287/3(cfblk14) -> cfblk366/1
  cfblk366/1 -> cfblk338/3(cfblk7)
  cfblk333/2(cfblk16) -> cfblk367/1
  cfblk367/1 -> cfblk132/1
  cfblk333/3(cfblk17) -> cfblk368/1
  cfblk368/1 -> cfblk299/3(cfblk13)
  cfblk123/1 -> cfblk369/1
  cfblk369/1 -> cfblk299/2(cfblk12)
  cfblk313/2(cfblk14) -> cfblk370/1
  cfblk370/1 -> cfblk297/2(cfblk4)
  cfblk43/1 -> cfblk371/1
  cfblk371/1 -> cfblk304/1(cfblk1)
  cfblk372/1 -> cfblk334/2(cfblk6)
  cfblk373/1 -> cfblk305/3(cfblk10)
  cfblk334/2(cfblk7) -> cfblk374/1
  cfblk374/1 -> cfblk298/1(cfblk1)
  cfblk53/1 -> cfblk375/1
  cfblk375/1 -> cfblk313/2(cfblk13)
  cfblk339/3(cfblk15) -> cfblk376/1
  cfblk376/1 -> cfblk315/3(cfblk9)
  cfblk315/3(cfblk12) -> cfblk377/1
  cfblk377/1 -> cfblk295/2(cfblk10)
  cfblk295/1(cfblk2) -> cfblk378/1
  cfblk378/1 -> cfblk290/1(cfblk1)
  cfblk321/3(cfblk8) -> cfblk379/1
  cfblk379/1 -> cfblk298/2(cfblk8)
  cfblk3/1 -> cfblk380/1
  cfblk380/1 -> cfblk312/2(cfblk10)
  cfblk311/3(cfblk13) -> cfblk381/1
  cfblk381/1 -> cfblk294/1(cfblk1)
  cfblk300/5(cfblk16) -> cfblk382/1
  cfblk382/1 -> cfblk127/1
  cfblk329/2(cfblk11) -> cfblk383/1
  cfblk383/1 -> cfblk319/2(cfblk14)
  cfblk329/4(cfblk13) -> cfblk384/1
  cfblk384/1 -> cfblk257/1
  cfblk200/1 -> cfblk385/1
  cfblk385/1 -> cfblk113/1

== system original/cfblk204 ==
  Demux : Demux  Tag=STV Demux  Outputs=1
  FromWs : FromWorkspace  Tag=STV FromWs  VariableName=tuvar  SampleTime=0
      SigBuilderData=|
      | common.afterFinalStr = 'Extrapolate'
      | common.sampleTime = 0
      | dataSet.timeRange = [0 10]
      | dataSet.name = 'Group 1'
      | sbobj.Groups.Name = 'Group 1'
      | sbobj.Groups.Signals.Name = 'Signal 1'
      | sbobj.Groups.Signals.XData = [0 4 4 6 6 10]
      | sbobj.Groups.Signals.YData = [0 0 1 1 0 0]
  Signal 1 : Outport  Tag=STV Outport
  wires:
  Demux/1 -> Signal 1/1
  FromWs/1 -> Demux/1

== system original/cfblk228 ==
  Demux : Demux  Tag=STV Demux  Outputs=1
  FromWs : FromWorkspace  Tag=STV FromWs  VariableName=tuvar  SampleTime=0
      SigBuilderData=|
      | common.afterFinalStr = 'Extrapolate'
      | common.sampleTime = 0
      | dataSet.timeRange = [0 10]
      | dataSet.name = 'Group 1'
      | sbobj.Groups.Name = 'Group 1'
      | sbobj.Groups.Signals.Name = 'Signal 1'
      | sbobj.Groups.Signals.XData = [0 4 4 6 6 10]
      | sbobj.Groups.Signals.YData = [0 0 1 1 0 0]
  Signal 1 : Outport  Tag=STV Outport
  wires:
  Demux/1 -> Signal 1/1
  FromWs/1 -> Demux/1

== system original/cfblk242 ==
  Demux : Demux  Tag=STV Demux  Outputs=1
  FromWs : FromWorkspace  Tag=STV FromWs  VariableName=tuvar  SampleTime=0
      SigBuilderData=|
      | common.afterFinalStr = 'Extrapolate'
      | common.sampleTime = 0
      | dataSet.timeRange = [0 10]
      | dataSet.name = 'Group 1'
      | sbobj.Groups.Name = 'Group 1'
      | sbobj.Groups.Signals.Name = 'Signal 1'
      | sbobj.Groups.Signals.XData = [0 4 4 6 6 10]
      | sbobj.Groups.Signals.YData = [0 0 1 1 0 0]
  Signal 1 : Outport  Tag=STV Outport
  wires:
  Demux/1 -> Signal 1/1
  FromWs/1 -> Demux/1

== system original/cfblk285 ==
  cfblk1 : Inport
  cfblk11 : Inport  Port=2
  Action Port : ActionPort  ActionType=then
  cfblk10 : DiscreteTransferFcn
  cfblk13 : Delay
  cfblk3 : DiscreteZeroPole  Poles=[0 0.5]  Gain=1  SampleTime=-1
  cfblk4 : simulink/Discrete/Tapped Delay  vinit=0.0  samptime=-1  NumDelays=1  DelayOrder=Oldest  includeCurrent=off
  cfblk5 : DiscreteTransferFcn
  cfblk6 : simulink/Continuous/PID Controller (2DOF)  Controller=PID  TimeDomain=Discrete-time  SampleTime=-1  IntegratorMethod=Forward Euler  FilterMethod=Forward Euler  Form=Parallel  UseFilter=on  ControllerParametersSource=internal  P=1  I=1  D=0  N=100  b=1  c=1  InitialConditionSource=internal  InitialConditionForIntegrator=0  InitialConditionForFilter=0  ExternalReset=none  LimitOutput=off  UpperSaturationLimit=inf  LowerSaturationLimit=-inf  LinearizeAsGain=off  AntiWindupMode=none  Kb=1  TrackingMode=off  Kt=1  PParamMin=[]  PParamMax=[]  IParamMin=[]  IParamMax=[]  DParamMin=[]  DParamMax=[]  NParamMin=[]  NParamMax=[]  bParamMin=[]  bParamMax=[]  cParamMin=[]  cParamMax=[]  KbParamMin=[]  KbParamMax=[]  KtParamMin=[]  KtParamMax=[]  POutMin=[]  POutMax=[]  IOutMin=[]  IOutMax=[]  DOutMin=[]  DOutMax=[]  NOutMin=[]  NOutMax=[]  bOutMin=[]  bOutMax=[]  cOutMin=[]  cOutMax=[]  KbOutMin=[]  KbOutMax=[]  KtOutMin=[]  KtOutMax=[]  IntegratorOutMin=[]  IntegratorOutMax=[]  FilterOutMin=[]  FilterOutMax=[]  SumOutMin=[]  SumOutMax=[]  Sum1OutMin=[]  Sum1OutMax=[]  Sum2OutMin=[]  Sum2OutMax=[]  Sum3OutMin=[]  Sum3OutMax=[]  SumI1OutMin=[]  SumI1OutMax=[]  SumI2OutMin=[]  SumI2OutMax=[]  SumI3OutMin=[]  SumI3OutMax=[]  SumDOutMin=[]  SumDOutMax=[]  SaturationOutMin=[]  SaturationOutMax=[]  IntegratorContinuousStateAttributes=''  IntegratorStateMustResolveToSignalObject=off  IntegratorRTWStateStorageClass=Auto  FilterContinuousStateAttributes=''  FilterStateMustResolveToSignalObject=off  FilterRTWStateStorageClass=Auto  DifferentiatorICPrevScaledInput=0  DifferentiatorOutMin=[]  DifferentiatorOutMax=[]  FilterDiffOutCoefMin=[]  FilterDiffOutCoefMax=[]  SumDenOutMin=[]  SumDenOutMax=[]  SumNumOutMin=[]  SumNumOutMax=[]  ReciprocalOutMin=[]  ReciprocalOutMax=[]  DivideOutMin=[]  DivideOutMax=[]  TunerSelectOption=Transfer Function Based (PID Tuner App)
  cfblk7 : DiscreteFilter
  cfblk8 : simulink/Discrete/Transfer Fcn Lead or Lag  PoleZ=0.95  ZeroZ=0.75  ICPrevOutput=0.0  ICPrevInput=0.0  DoSatur=off
      settings: SourceProductName=Simulink  SourceProductBaseCode=SL
  cfblk9 : simulink/Continuous/PID Controller  Controller=PID  TimeDomain=Discrete-time  SampleTime=-1  IntegratorMethod=Forward Euler  FilterMethod=Forward Euler  Form=Parallel  UseFilter=on  ControllerParametersSource=internal  P=1  I=1  D=0  N=100  InitialConditionSource=internal  InitialConditionForIntegrator=0  InitialConditionForFilter=0  ExternalReset=none  LimitOutput=off  UpperSaturationLimit=inf  LowerSaturationLimit=-inf  LinearizeAsGain=off  AntiWindupMode=none  Kb=1  TrackingMode=off  Kt=1  PParamMin=[]  PParamMax=[]  IParamMin=[]  IParamMax=[]  DParamMin=[]  DParamMax=[]  NParamMin=[]  NParamMax=[]  KbParamMin=[]  KbParamMax=[]  KtParamMin=[]  KtParamMax=[]  POutMin=[]  POutMax=[]  IOutMin=[]  IOutMax=[]  DOutMin=[]  DOutMax=[]  NOutMin=[]  NOutMax=[]  KbOutMin=[]  KbOutMax=[]  KtOutMin=[]  KtOutMax=[]  IntegratorOutMin=[]  IntegratorOutMax=[]  FilterOutMin=[]  FilterOutMax=[]  SumOutMin=[]  SumOutMax=[]  SumI1OutMin=[]  SumI1OutMax=[]  SumI2OutMin=[]  SumI2OutMax=[]  SumI3OutMin=[]  SumI3OutMax=[]  SumDOutMin=[]  SumDOutMax=[]  SaturationOutMin=[]  SaturationOutMax=[]  IntegratorContinuousStateAttributes=''  IntegratorStateMustResolveToSignalObject=off  IntegratorRTWStateStorageClass=Auto  FilterContinuousStateAttributes=''  FilterStateMustResolveToSignalObject=off  FilterRTWStateStorageClass=Auto  DifferentiatorICPrevScaledInput=0  DifferentiatorOutMin=[]  DifferentiatorOutMax=[]  FilterDiffOutCoefMin=[]  FilterDiffOutCoefMax=[]  SumDenOutMin=[]  SumDenOutMax=[]  SumNumOutMin=[]  SumNumOutMax=[]  ReciprocalOutMin=[]  ReciprocalOutMax=[]  DivideOutMin=[]  DivideOutMax=[]  TunerSelectOption=Transfer Function Based (PID Tuner App)
  cfblk2 : Outport
  cfblk12 : Outport  Port=2
  wires:
  cfblk3/1 -> cfblk5/1, cfblk10/1
  cfblk9/1 -> cfblk6/1
  cfblk6/1 -> cfblk12/1
  cfblk10/1 -> cfblk8/1
  cfblk4/1 -> cfblk6/2
  cfblk11/1 -> cfblk2/1
  cfblk7/1 -> cfblk4/1
  cfblk1/1 -> cfblk9/1
  cfblk5/1 -> cfblk7/1
  cfblk8/1 -> cfblk13/1
  cfblk13/1 -> cfblk3/1

== system original/cfblk286 ==
  cfblk1 : Inport
  Action Port : ActionPort  ActionType=else
  cfblk11 : Subsystem  TreatAsAtomicUnit=on
  cfblk12 : Subsystem  TreatAsAtomicUnit=on
  cfblk13 : Delay
  cfblk14 : Delay
  cfblk15 : Delay
  cfblk3 : DiscreteFir
  cfblk4 : simulink/Discrete/Transfer Fcn Real Zero  ZeroZ=0.75  ICPrevInput=0.0  DoSatur=off
      settings: SourceProductName=Simulink  SourceProductBaseCode=SL
  cfblk5 : DiscreteZeroPole  Poles=[0 0.5]  Gain=1  SampleTime=-1
  cfblk6 : simulink/Discrete/Difference  ICPrevInput=0.0  OutMin=[]  OutMax=[]  OutDataTypeStr=Inherit: Inherit via back propagation  OutDataType=fixdt(1, 16)  OutScaling=2^-10  DoSatur=off
  cfblk7 : Delay  ShowEnablePort=on
      settings: InputPortMap=u0,e6
  cfblk8 : DiscreteFir
  cfblk9 : If  SampleTime=1
  cfblk2 : Outport
  cfblk10 : Outport  Port=2
  wires:
  cfblk6/1 -> cfblk2/1
  cfblk3/1 -> cfblk5/1
  cfblk11/1(cfblk2) -> cfblk4/1
  cfblk8/1 -> cfblk14/1, cfblk15/1
  cfblk5/1 -> cfblk6/1, cfblk13/1
  cfblk7/1 -> cfblk3/1
  cfblk11/2(cfblk9) -> cfblk10/1
  cfblk12/1(cfblk2) -> cfblk11/1(cfblk1), cfblk8/1, cfblk7/2
  cfblk4/1 -> cfblk7/1
  cfblk1/1 -> cfblk12/1(cfblk1)
  cfblk9/1 -> cfblk11/Action
  cfblk9/2 -> cfblk12/Action
  cfblk13/1 -> cfblk12/2(cfblk16)
  cfblk14/1 -> cfblk9/1
  cfblk15/1 -> cfblk12/3(cfblk17)

== system original/cfblk287 ==
  cfblk1 : Inport
  cfblk12 : Inport  Port=2
  Action Port : ActionPort  ActionType=then
  cfblk10 : DiscreteTransferFcn
  cfblk11 : If  SampleTime=1
  cfblk15 : Subsystem  TreatAsAtomicUnit=on
  cfblk16 : Subsystem  TreatAsAtomicUnit=on
  cfblk{9,17..19} (4 alike) : Delay
  cfblk3 : Delay  DelayLengthSource=Input port
      settings: InputPortMap=u0,p1
  cfblk4 : simulink/Discrete/Transfer Fcn First Order  PoleZ=0.95  ICPrevOutput=0.0  DoSatur=off
      settings: SourceProductName=Simulink
  cfblk5 : DiscreteIntegrator  SampleTime=-1  ICPrevOutput=DiscIntNeverNeededParam  ICPrevScaledInput=DiscIntNeverNeededParam
  cfblk6 : simulink/Discrete/Transfer Fcn Real Zero  ZeroZ=0.75  ICPrevInput=0.0  DoSatur=off
      settings: SourceProductName=Simulink  SourceProductBaseCode=SL
  cfblk7 : Delay  ShowEnablePort=on
      settings: InputPortMap=u0,e6
  cfblk8 : simulink/Discrete/Transfer Fcn Real Zero  ZeroZ=0.75  ICPrevInput=0.0  DoSatur=off
      settings: SourceProductName=Simulink  SourceProductBaseCode=SL
  cfblk2 : Outport
  cfblk13 : Outport  Port=2
  cfblk14 : Outport  Port=3
  wires:
  cfblk4/1 -> cfblk2/1
  cfblk15/1(cfblk2) -> cfblk4/1
  cfblk16/1(cfblk2) -> cfblk8/1
  cfblk3/1 -> cfblk7/1
  cfblk9/1 -> cfblk6/1
  cfblk12/1 -> cfblk5/1
  cfblk5/1 -> cfblk7/2
  cfblk16/2(cfblk13) -> cfblk9/1
  cfblk7/1 -> cfblk14/1, cfblk16/2(cfblk12)
  cfblk15/3(cfblk12) -> cfblk13/1
  cfblk1/1 -> cfblk10/1
  cfblk10/1 -> cfblk3/2, cfblk16/1(cfblk1)
  cfblk11/1 -> cfblk15/Action
  cfblk11/2 -> cfblk16/Action
  cfblk8/1 -> cfblk17/1
  cfblk17/1 -> cfblk15/1(cfblk1)
  cfblk15/2(cfblk11) -> cfblk18/1
  cfblk18/1 -> cfblk3/1
  cfblk6/1 -> cfblk19/1
  cfblk19/1 -> cfblk11/1

== system original/cfblk288 ==
  cfblk1 : Inport
  cfblk7 : Inport  Port=2
  Action Port : ActionPort  ActionType=else
  cfblk3 : DiscreteStateSpace  SampleTime=-1
  cfblk4 : simulink/Discrete/Transfer Fcn Real Zero  ZeroZ=0.75  ICPrevInput=0.0  DoSatur=off
      settings: SourceProductName=Simulink  SourceProductBaseCode=SL
  cfblk5 : simulink/Continuous/PID Controller (2DOF)  Controller=PID  TimeDomain=Discrete-time  SampleTime=-1  IntegratorMethod=Forward Euler  FilterMethod=Forward Euler  Form=Parallel  UseFilter=on  ControllerParametersSource=internal  P=1  I=1  D=0  N=100  b=1  c=1  InitialConditionSource=internal  InitialConditionForIntegrator=0  InitialConditionForFilter=0  ExternalReset=none  LimitOutput=off  UpperSaturationLimit=inf  LowerSaturationLimit=-inf  LinearizeAsGain=off  AntiWindupMode=none  Kb=1  TrackingMode=off  Kt=1  PParamMin=[]  PParamMax=[]  IParamMin=[]  IParamMax=[]  DParamMin=[]  DParamMax=[]  NParamMin=[]  NParamMax=[]  bParamMin=[]  bParamMax=[]  cParamMin=[]  cParamMax=[]  KbParamMin=[]  KbParamMax=[]  KtParamMin=[]  KtParamMax=[]  POutMin=[]  POutMax=[]  IOutMin=[]  IOutMax=[]  DOutMin=[]  DOutMax=[]  NOutMin=[]  NOutMax=[]  bOutMin=[]  bOutMax=[]  cOutMin=[]  cOutMax=[]  KbOutMin=[]  KbOutMax=[]  KtOutMin=[]  KtOutMax=[]  IntegratorOutMin=[]  IntegratorOutMax=[]  FilterOutMin=[]  FilterOutMax=[]  SumOutMin=[]  SumOutMax=[]  Sum1OutMin=[]  Sum1OutMax=[]  Sum2OutMin=[]  Sum2OutMax=[]  Sum3OutMin=[]  Sum3OutMax=[]  SumI1OutMin=[]  SumI1OutMax=[]  SumI2OutMin=[]  SumI2OutMax=[]  SumI3OutMin=[]  SumI3OutMax=[]  SumDOutMin=[]  SumDOutMax=[]  SaturationOutMin=[]  SaturationOutMax=[]  IntegratorContinuousStateAttributes=''  IntegratorStateMustResolveToSignalObject=off  IntegratorRTWStateStorageClass=Auto  FilterContinuousStateAttributes=''  FilterStateMustResolveToSignalObject=off  FilterRTWStateStorageClass=Auto  DifferentiatorICPrevScaledInput=0  DifferentiatorOutMin=[]  DifferentiatorOutMax=[]  FilterDiffOutCoefMin=[]  FilterDiffOutCoefMax=[]  SumDenOutMin=[]  SumDenOutMax=[]  SumNumOutMin=[]  SumNumOutMax=[]  ReciprocalOutMin=[]  ReciprocalOutMax=[]  DivideOutMin=[]  DivideOutMax=[]  TunerSelectOption=Transfer Function Based (PID Tuner App)
  cfblk6 : Delay  ShowEnablePort=on
      settings: InputPortMap=u0,e6
  cfblk2 : Outport
  cfblk8 : Outport  Port=2
  cfblk9 : Outport  Port=3
  wires:
  cfblk5/1 -> cfblk6/1
  cfblk6/1 -> cfblk2/1
  cfblk1/1 -> cfblk3/1
  cfblk3/1 -> cfblk5/1, cfblk8/1
  cfblk7/1 -> cfblk5/2, cfblk4/1, cfblk9/1
  cfblk4/1 -> cfblk6/2

== system original/cfblk289 ==
  cfblk1 : Inport
  cfblk6 : Inport  Port=2
  Action Port : ActionPort  ActionType=then
  cfblk3 : DiscreteZeroPole  Poles=[0 0.5]  Gain=1  SampleTime=-1
  cfblk4 : DiscreteFilter
  cfblk5 : DiscreteStateSpace  SampleTime=-1
  cfblk2 : Outport
  cfblk7 : Outport  Port=2
  wires:
  cfblk6/1 -> cfblk5/1
  cfblk4/1 -> cfblk2/1
  cfblk5/1 -> cfblk3/1
  cfblk1/1 -> cfblk7/1
  cfblk3/1 -> cfblk4/1

== system original/cfblk290 ==
  cfblk1 : Inport
  cfblk9 : Inport  Port=2
  cfblk10 : Inport  Port=3
  Action Port : ActionPort  ActionType=else
  cfblk12 : Delay
  cfblk3 : DiscreteZeroPole  Poles=[0 0.5]  Gain=1  SampleTime=-1
  cfblk4 : simulink/Discrete/Tapped Delay  vinit=0.0  samptime=-1  NumDelays=1  DelayOrder=Oldest  includeCurrent=off
  cfblk5 : Delay  ShowEnablePort=on
      settings: InputPortMap=u0,e6
  cfblk6 : simulink/Continuous/PID Controller (2DOF)  Controller=PID  TimeDomain=Discrete-time  SampleTime=-1  IntegratorMethod=Forward Euler  FilterMethod=Forward Euler  Form=Parallel  UseFilter=on  ControllerParametersSource=internal  P=1  I=1  D=0  N=100  b=1  c=1  InitialConditionSource=internal  InitialConditionForIntegrator=0  InitialConditionForFilter=0  ExternalReset=none  LimitOutput=off  UpperSaturationLimit=inf  LowerSaturationLimit=-inf  LinearizeAsGain=off  AntiWindupMode=none  Kb=1  TrackingMode=off  Kt=1  PParamMin=[]  PParamMax=[]  IParamMin=[]  IParamMax=[]  DParamMin=[]  DParamMax=[]  NParamMin=[]  NParamMax=[]  bParamMin=[]  bParamMax=[]  cParamMin=[]  cParamMax=[]  KbParamMin=[]  KbParamMax=[]  KtParamMin=[]  KtParamMax=[]  POutMin=[]  POutMax=[]  IOutMin=[]  IOutMax=[]  DOutMin=[]  DOutMax=[]  NOutMin=[]  NOutMax=[]  bOutMin=[]  bOutMax=[]  cOutMin=[]  cOutMax=[]  KbOutMin=[]  KbOutMax=[]  KtOutMin=[]  KtOutMax=[]  IntegratorOutMin=[]  IntegratorOutMax=[]  FilterOutMin=[]  FilterOutMax=[]  SumOutMin=[]  SumOutMax=[]  Sum1OutMin=[]  Sum1OutMax=[]  Sum2OutMin=[]  Sum2OutMax=[]  Sum3OutMin=[]  Sum3OutMax=[]  SumI1OutMin=[]  SumI1OutMax=[]  SumI2OutMin=[]  SumI2OutMax=[]  SumI3OutMin=[]  SumI3OutMax=[]  SumDOutMin=[]  SumDOutMax=[]  SaturationOutMin=[]  SaturationOutMax=[]  IntegratorContinuousStateAttributes=''  IntegratorStateMustResolveToSignalObject=off  IntegratorRTWStateStorageClass=Auto  FilterContinuousStateAttributes=''  FilterStateMustResolveToSignalObject=off  FilterRTWStateStorageClass=Auto  DifferentiatorICPrevScaledInput=0  DifferentiatorOutMin=[]  DifferentiatorOutMax=[]  FilterDiffOutCoefMin=[]  FilterDiffOutCoefMax=[]  SumDenOutMin=[]  SumDenOutMax=[]  SumNumOutMin=[]  SumNumOutMax=[]  ReciprocalOutMin=[]  ReciprocalOutMax=[]  DivideOutMin=[]  DivideOutMax=[]  TunerSelectOption=Transfer Function Based (PID Tuner App)
  cfblk7 : simulink/Discrete/Difference  ICPrevInput=0.0  OutMin=[]  OutMax=[]  OutDataTypeStr=Inherit: Inherit via back propagation  OutDataType=fixdt(1, 16)  OutScaling=2^-10  DoSatur=off
  cfblk8 : DiscreteIntegrator  SampleTime=-1  ICPrevOutput=DiscIntNeverNeededParam  ICPrevScaledInput=DiscIntNeverNeededParam
  cfblk2 : Outport
  cfblk11 : Outport  Port=2
  wires:
  cfblk3/1 -> cfblk5/1
  cfblk7/1 -> cfblk6/1
  cfblk4/1 -> cfblk7/1
  cfblk10/1 -> cfblk6/2, cfblk5/2
  cfblk1/1 -> cfblk8/1
  cfblk6/1 -> cfblk11/1
  cfblk9/1 -> cfblk2/1
  cfblk8/1 -> cfblk4/1
  cfblk5/1 -> cfblk12/1
  cfblk12/1 -> cfblk3/1

== system original/cfblk291 ==
  cfblk1 : Inport
  cfblk7 : Inport  Port=2
  Action Port : ActionPort  ActionType=then
  cfblk3 : simulink/Discrete/Tapped Delay  vinit=0.0  samptime=-1  NumDelays=1  DelayOrder=Oldest  includeCurrent=off
  cfblk4 : simulink/Continuous/PID Controller  Controller=PID  TimeDomain=Discrete-time  SampleTime=-1  IntegratorMethod=Forward Euler  FilterMethod=Forward Euler  Form=Parallel  UseFilter=on  ControllerParametersSource=internal  P=1  I=1  D=0  N=100  InitialConditionSource=internal  InitialConditionForIntegrator=0  InitialConditionForFilter=0  ExternalReset=none  LimitOutput=off  UpperSaturationLimit=inf  LowerSaturationLimit=-inf  LinearizeAsGain=off  AntiWindupMode=none  Kb=1  TrackingMode=off  Kt=1  PParamMin=[]  PParamMax=[]  IParamMin=[]  IParamMax=[]  DParamMin=[]  DParamMax=[]  NParamMin=[]  NParamMax=[]  KbParamMin=[]  KbParamMax=[]  KtParamMin=[]  KtParamMax=[]  POutMin=[]  POutMax=[]  IOutMin=[]  IOutMax=[]  DOutMin=[]  DOutMax=[]  NOutMin=[]  NOutMax=[]  KbOutMin=[]  KbOutMax=[]  KtOutMin=[]  KtOutMax=[]  IntegratorOutMin=[]  IntegratorOutMax=[]  FilterOutMin=[]  FilterOutMax=[]  SumOutMin=[]  SumOutMax=[]  SumI1OutMin=[]  SumI1OutMax=[]  SumI2OutMin=[]  SumI2OutMax=[]  SumI3OutMin=[]  SumI3OutMax=[]  SumDOutMin=[]  SumDOutMax=[]  SaturationOutMin=[]  SaturationOutMax=[]  IntegratorContinuousStateAttributes=''  IntegratorStateMustResolveToSignalObject=off  IntegratorRTWStateStorageClass=Auto  FilterContinuousStateAttributes=''  FilterStateMustResolveToSignalObject=off  FilterRTWStateStorageClass=Auto  DifferentiatorICPrevScaledInput=0  DifferentiatorOutMin=[]  DifferentiatorOutMax=[]  FilterDiffOutCoefMin=[]  FilterDiffOutCoefMax=[]  SumDenOutMin=[]  SumDenOutMax=[]  SumNumOutMin=[]  SumNumOutMax=[]  ReciprocalOutMin=[]  ReciprocalOutMax=[]  DivideOutMin=[]  DivideOutMax=[]  TunerSelectOption=Transfer Function Based (PID Tuner App)
  cfblk5 : DiscreteFilter
  cfblk6 : UnitDelay  SampleTime=-1
  cfblk2 : Outport
  cfblk8 : Outport  Port=2
  cfblk9 : Outport  Port=3
  wires:
  cfblk7/1 -> cfblk3/1
  cfblk5/1 -> cfblk2/1
  cfblk4/1 -> cfblk8/1
  cfblk3/1 -> cfblk9/1
  cfblk6/1 -> cfblk4/1
  cfblk1/1 -> cfblk5/1, cfblk6/1
